simulink model "G24i_v_source"  (R2014a)
settings: Solver=ode23tb  StartTime=0.0  StopTime=5  RelTol=1e-4
values from neighbouring files (symbols this model uses):
  Array_Voc = [0.328644000009 2.76811 3.09396940822 3.26133568944 3.36629977409 3.44398192097 3.50365713438 3.55225637345 3.59363766529 3.63021764721 3.6624 3.69037314882 ... (101 elements, 101x1)]    [Array_Voc.mat]
  ArrayCurrent = [1.05303e-05 0.0329007487024 0.0659314357778 0.100205 0.132978217474 0.166891516648 0.200872978445 0.234107600227 0.267513340222 0.302009988541 0.336322 0.36979130469 ... (44440 elements, 101x440)]    [ArrayCurrent.mat]    (also in Genrate_SC_mod.m = fitresult_normal_g42(V,G); temp3.m = fitresult(V,G))
  ArrayVoltage = [0 0.01 0.02 0.03 0.04 0.05 0.06 0.07 0.08 0.09 0.1 0.11 ... (440 elements, 1x440)]    [ArrayVoltage.mat]    (also in Genrate_SC_mod.m = (0:0.01:max(Voltage)); temp3.m = (0:0.01:max(Voltage)))
  Irradiance = (min(Lux):50:max(Lux))    [Genrate_SC_mod.m]    (also in Irradiance.mat = [0 50 100 150 200 250 300 350 400 450 500 550 ... (101 eleme; temp3.m)
undefined symbols (not defined in the file or in its folder): sigbuilder_block
libraries: powerlib x7, simulink_extras x4
settings Model: NumberOfSteps=5  Creator=kartik.karuna  LastModifiedBy=kartik.karuna
settings SolverCC: SolverJacobianMethodControl=SparsePerturbation  ZeroCrossAlgorithm=Adaptive  AutoInsertRateTranBlk=on

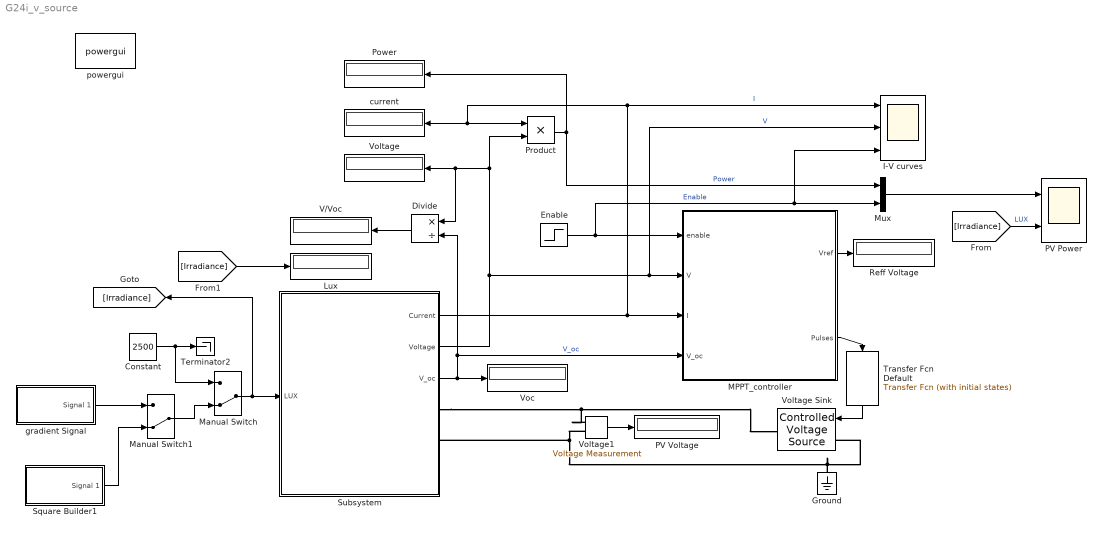
== system G24i_v_source ==
  Constant : Constant  Value=2500
  Divide : Product  Inputs=*/
  Enable : Step  Time=0.1  SampleTime=0
  Ground : powerlib/Elements/Ground  LConnTagsString=a
  I-V curves : Scope  NumInputPorts=3
      settings: ShowLegends=on  TimeRange=0.09  YMin=0.45~3.4875~1  YMax=0.8~3.5125~1
  Lux : Display
  MPPT_controller : Subsystem  Variant=on
  Manual Switch : ManualSwitch  CurrentSetting=0
  Manual Switch1 : ManualSwitch  CurrentSetting=0
  Mux : Mux  Inputs=2
  PV Power : Scope  NumInputPorts=2
      settings: ShowLegends=on  TimeRange=0.5  YMin=0~800  YMax=7~2000  SaveName=ScopeData2
  PV Voltage : Display
  Power : Display
  Product : Product  RndMeth=Zero
  Reff Voltage : Display
  Square Builder1 : Subsystem  Tag=STV Subsys  LoadFcn=sigbuilder_block('load');  StartFcn=sigbuilder_block('start');  StopFcn=sigbuilder_block('stop');  ClipboardFcn=sigbuilder_block('clipboard');  mask(Sigbuilder block){}
      mask help: Simulink:masks:SigbuilderBlock_MD
      mask init:
      | if ~strcmp(get_param(bdroot(gcbh),'SimulationStatus'),'stopped') tuvar = sigbuilder_block('maskInit'); end
      settings: CopyFcn=sigbuilder_block('copy');  DeleteFcn=sigbuilder_block('delete');  ModelCloseFcn=sigbuilder_block('modelClose');  PreSaveFcn=sigbuilder_block('preSave');  PauseFcn=sigbuilder_block('pause');  ContinueFcn=sigbuilder_block('continue');  NameChangeFcn=sigbuilder_block('namechange');  OpenFcn=sigbuilder_block('open',[0 29.7931 1588.97 810.621 ]);  CloseFcn=sigbuilder_block('close');
      mask Display: plot(0, 0, 100, 100,[2, 2, 32, 32, 2], [68, 8, 8, 68, 68],[32, 2], [38, 38], [32, 19, 2],[53, 60, 44], [32, 17, 17, 2],[16, 16, 31, 31]);txt = getActiveGroup(gcbh);text(2, 100, txt,'verticalAlignment', 'top');
  Subsystem : Subsystem
  Terminator2 : Terminator
  Transfer Fcn Default : simulink_extras/Additional Linear/Transfer Fcn (with initial states)  VariantControl=(default)  N=[1]  D="[.00001  1]"  X0=0
  V/Voc : Display
  Voc : Display
  Voltage : Display
  Voltage Sink : powerlib/Electrical Sources/Controlled Voltage Source  Initialize=on  Source_Type=AC  Amplitude=0  Phase=0  Frequency=0  Measurements=Voltage
  Voltage1 : powerlib/Measurements/Voltage Measurement  PhasorSimulation=off  OutputType=Complex  PSBequivalent=0
  current : Display
  gradient Signal : Subsystem  Tag=STV Subsys  LoadFcn=sigbuilder_block('load');  StartFcn=sigbuilder_block('start');  StopFcn=sigbuilder_block('stop');  ClipboardFcn=sigbuilder_block('clipboard');  mask(Sigbuilder block){}
      mask help: Simulink:masks:SigbuilderBlock_MD
      mask init:
      | if ~strcmp(get_param(bdroot(gcbh),'SimulationStatus'),'stopped') tuvar = sigbuilder_block('maskInit'); end
      settings: CopyFcn=sigbuilder_block('copy');  DeleteFcn=sigbuilder_block('delete');  ModelCloseFcn=sigbuilder_block('modelClose');  PreSaveFcn=sigbuilder_block('preSave');  PauseFcn=sigbuilder_block('pause');  ContinueFcn=sigbuilder_block('continue');  NameChangeFcn=sigbuilder_block('namechange');  OpenFcn=sigbuilder_block('open',[1588.97 178.759 1271.17 661.655 ]);  CloseFcn=sigbuilder_block('close');
      mask Display: plot(0, 0, 100, 100,[2, 2, 32, 32, 2], [68, 8, 8, 68, 68],[32, 2], [38, 38], [32, 19, 2],[53, 60, 44], [32, 17, 17, 2],[16, 16, 31, 31]);txt = getActiveGroup(gcbh);text(2, 100, txt,'verticalAlignment', 'top');
  powergui : powerlib/powergui  Priority=1  SimulationMode=Continuous  SolverType=Tustin  SampleTime=50e-6  frequency=50  SPID=off  DisableSnubberDevices=off  DisableRonSwitches=off  DisableVfSwitches=off  SwTol=0  Interpol=off  DisplayEquations=off  Ts=0  methode=off  frequencyindice=0  Pbase=100e6  ErrMax=1e-4  Iterations=50  UnitsV=kV  UnitsW=MW  FunctionMessages=off  echomessages=off  HookPort=off  EnableUseOfTLC=off  x0status=blocks  RestoreLinks=warning  ResistiveCurrentMeasurement=off  Frange=[0:2:500]  Ylog=off  Xlog=on  ShowGrid=off  save=off  variable=ZData  structure=0  ZoomFFT=off  StartTime=0.0  cycles=1  DisplayStyle=1  fundamental=60  FreqAxis=off  MaxFrequency=1000  frequencyindicesteady=1  RmsSteady=1  display=off
  wires:
  Mux/1 -> PV Power/1
  Product/1 -> Power/1, Mux/1  "Power"
  Voltage1/1 -> PV Voltage/1
  Enable/1 -> MPPT_controller/1(enable), I-V curves/3, Mux/2  "Enable"
  Subsystem/3("V_oc ") -> Divide/2, MPPT_controller/4(V_oc), Voc/1  "V_oc"
  Divide/1 -> V/Voc/1
  MPPT_controller/1(Vref) -> Reff Voltage/1
  Subsystem/2(Voltage) -> Divide/1, Voltage/1, Product/2, I-V curves/2, MPPT_controller/2(V)  "V"
  Subsystem/1(Current) -> I-V curves/1, current/1, Product/1, MPPT_controller/3(I)  "I"
  Constant/1 -> Manual Switch/1, Terminator2/1
  [Irradiance] -> PV Power/2  "LUX"
  Manual Switch/1 -> Subsystem/1(LUX), [Irradiance]
  [Irradiance] -> Lux/1
  Manual Switch1/1 -> Manual Switch/2
  gradient Signal/1(Signal 1) -> Manual Switch1/1
  Square Builder1/1(Signal 1) -> Manual Switch1/2
  MPPT_controller/2(Pulses) -> Transfer Fcn Default/1
  Transfer Fcn Default/1 -> Voltage Sink/1
  connections:
  Subsystem/RConn1 -- Voltage1/LConn1 -- Voltage Sink/RConn1
  Voltage1/LConn2 -- Voltage Sink/LConn1 -- Ground/LConn1 -- Subsystem/RConn2

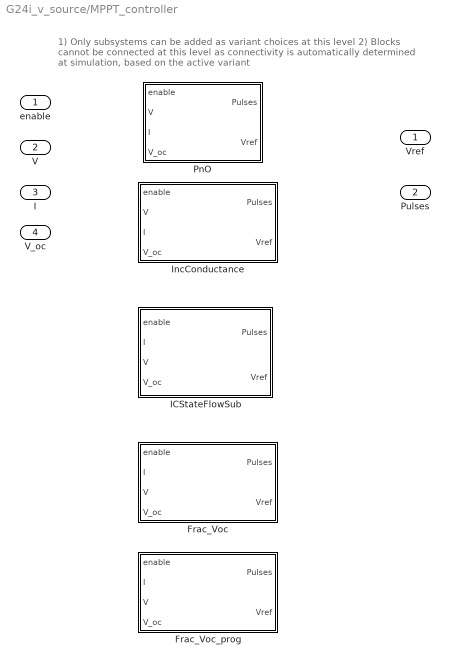
== system G24i_v_source/MPPT_controller ==
  note: 1) Only subsystems can be added as variant choices at this level
      | 2) Blocks cannot be connected at this level as connectivity is
      | automatically determined at simulation, based on the active variant
  enable : Inport
  V : Inport  Port=2
  I : Inport  Port=3
  V_oc : Inport  Port=4
  Frac_Voc : Subsystem  VariantControl=MPPT_Frac_Voc
  Frac_Voc_prog : Subsystem  VariantControl=MPPT_Frac_Voc_prog
  ICStateFlowSub : Subsystem  VariantControl=MPPT_IC_SF
  IncConductance : Subsystem  VariantControl=MPPT_IC_logic
  PnO : Subsystem  VariantControl=MPPT_PnO
  Vref : Outport
  Pulses : Outport  Port=2

== system G24i_v_source/Square Builder1 ==
  Demux : Demux  Tag=STV Demux  Outputs=1
  FromWs : FromWorkspace  Tag=STV FromWs  VariableName=tuvar  SampleTime=0
      SigBuilderData=|
      | common.afterFinalStr = 'Extrapolate'
      | common.sampleTime = 0
      | dataSet.timeRange = [0 2]
      | dataSet.name = 'Group 1'
      | sbobj.Groups.Name = 'Group 1'
      | sbobj.Groups.Signals.Name = 'Signal 1'
      | sbobj.Groups.Signals.XData = [0 0.3 0.4 0.4 0.6 0.6 0.6 0.7 0.7 0.8 0.8 1.1 1.1 1.2 1.2 1.4 1.4 1.8 1.8 1.9 2]
      | sbobj.Groups.Signals.YData = [2500 2500 2500 2000 2000 1500 1500 1500 1000 1000 800 800 1200 1200 1500 1500 1000 1000 400 400 400]
      | sbobj.Groups.TimeRange = [0 2]
  Signal 1 : Outport  Tag=STV Outport
  wires:
  FromWs/1 -> Demux/1
  Demux/1 -> Signal 1/1

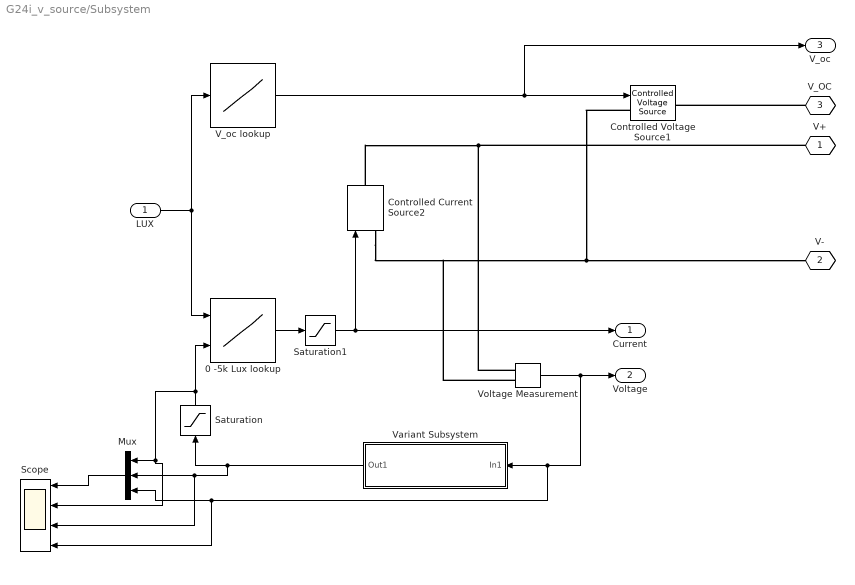
== system G24i_v_source/Subsystem ==
  LUX : Inport
  0 -5k Lux lookup : Lookup_n-D  BreakpointsForDimension1=Irradiance  BreakpointsForDimension2=ArrayVoltage  BreakpointsForDimension1Min=[0]  BreakpointsForDimension2Min=[0]  BreakpointsForDimension1Max=[5000]  BreakpointsForDimension2Max=[6]  Table=ArrayCurrent  DiagnosticForOutOfRangeInput=Warning  RndMeth=Simplest  InputSameDT=on
  Controlled Current Source2 : powerlib/Electrical Sources/Controlled Current Source  Initialize=on  Source_Type=DC  Amplitude=0  Phase=0  Frequency=0  Measurements=None
  Controlled Voltage Source1 : powerlib/Electrical Sources/Controlled Voltage Source  Initialize=on  Source_Type=AC  Amplitude=0  Phase=0  Frequency=0  Measurements=Voltage
  Mux : Mux  Inputs=3
  Saturation : Saturate  UpperLimit=6  LowerLimit=0  ZeroCross=off
  Saturation1 : Saturate  UpperLimit=6  LowerLimit=-1
  Scope : Scope  NumInputPorts=4
      settings: YMin=-5~-5~-5~-5  YMax=5~5~5~5
  V_oc lookup : Lookup_n-D  NumberOfTableDimensions=1  BreakpointsForDimension1=Irradiance  Table=Array_Voc  RndMeth=Simplest  InputSameDT=on
  Variant Subsystem : Subsystem  Variant=on
  Voltage Measurement : powerlib/Measurements/Voltage Measurement  PhasorSimulation=off  OutputType=Complex  PSBequivalent=0
  V+ : PMIOPort  Tag=PMCPort  Port=1  Side=Right
  V- : PMIOPort  Tag=PMCPort  Port=2  Side=Right
  V_OC : PMIOPort  Tag=PMCPort  Port=3  Side=Right
  Current : Outport
  Voltage : Outport  Port=2
  "V_oc " : Outport  Port=3
  wires:
  LUX/1 -> 0 -5k Lux lookup/1, V_oc lookup/1
  Voltage Measurement/1 -> Voltage/1, Scope/4, Mux/3, Variant Subsystem/1(In1)
  0 -5k Lux lookup/1 -> Saturation1/1
  V_oc lookup/1 -> "V_oc "/1, Controlled Voltage Source1/1
  Saturation/1 -> 0 -5k Lux lookup/2, Scope/2, Mux/1
  Saturation1/1 -> Controlled Current Source2/1, Current/1
  Mux/1 -> Scope/1
  Variant Subsystem/1(Out1) -> Scope/3, Mux/2, Saturation/1
  connections:
  Controlled Current Source2/RConn1 -- V+/RConn1 -- Voltage Measurement/LConn1
  Controlled Voltage Source1/LConn1 -- Voltage Measurement/LConn2 -- Controlled Current Source2/LConn1 -- V-/RConn1
  V_OC/RConn1 -- Controlled Voltage Source1/RConn1

== system G24i_v_source/gradient Signal ==
  Demux : Demux  Tag=STV Demux  Outputs=1
  FromWs : FromWorkspace  Tag=STV FromWs  VariableName=tuvar  SampleTime=0
      SigBuilderData=|
      | common.afterFinalStr = 'Extrapolate'
      | common.sampleTime = 0
      | dataSet.timeRange = [0 2]
      | dataSet.name = 'Group 1'
      | sbobj.Groups.Name = 'Group 1'
      | sbobj.Groups.Signals.Name = 'Signal 1'
      | sbobj.Groups.Signals.XData = [0 0.35 0.55 0.85 1.2 2]
      | sbobj.Groups.Signals.YData = [2500 2500 200 200 800 800]
      | sbobj.Groups.TimeRange = [0 2]
  Signal 1 : Outport  Tag=STV Outport
  wires:
  Demux/1 -> Signal 1/1
  FromWs/1 -> Demux/1

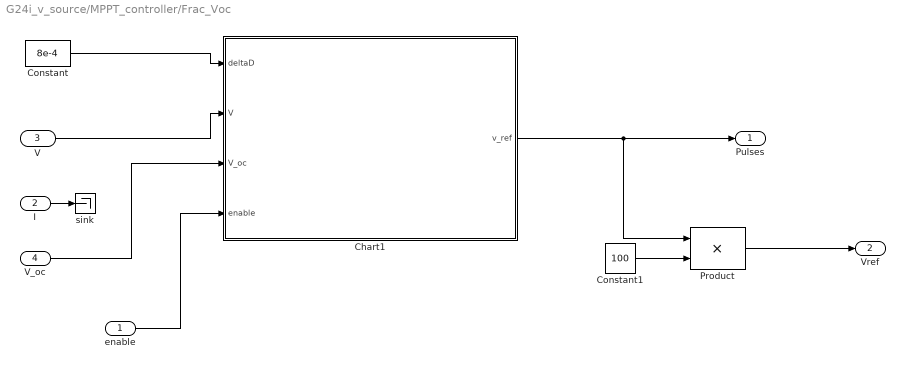
== system G24i_v_source/MPPT_controller/Frac_Voc ==
  enable : Inport
  I : Inport  Port=2
  V : Inport  Port=3
  V_oc : Inport  Port=4
  Chart1 : Stateflow chart  TreatAsAtomicUnit=on
  Constant : Constant  Value=8e-4
  Constant1 : Constant  Value=100
  Product : Product  RndMeth=Zero
  sink : Terminator
  Pulses : Outport
  Vref : Outport  Port=2
  wires:
  Constant/1 -> Chart1/1(deltaD)
  V/1 -> Chart1/2(V)
  enable/1 -> Chart1/4(enable)
  Chart1/1(v_ref) -> Pulses/1, Product/1
  Constant1/1 -> Product/2
  Product/1 -> Vref/1
  V_oc/1 -> Chart1/3(V_oc)
  I/1 -> sink/1

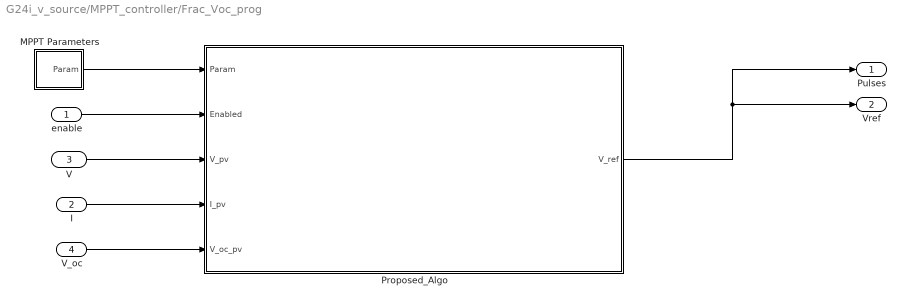
== system G24i_v_source/MPPT_controller/Frac_Voc_prog ==
  enable : Inport
  I : Inport  Port=2
  V : Inport  Port=3
  V_oc : Inport  Port=4
  MPPT Parameters : Subsystem
  Proposed_Algo : MATLAB Function  TreatAsAtomicUnit=on
  Pulses : Outport
  Vref : Outport  Port=2
  wires:
  I/1 -> Proposed_Algo/4(I_pv)
  MPPT Parameters/1(Param) -> Proposed_Algo/1(Param)
  enable/1 -> Proposed_Algo/2(Enabled)
  V/1 -> Proposed_Algo/3(V_pv)
  V_oc/1 -> Proposed_Algo/5(V_oc_pv)
  Proposed_Algo/1(V_ref) -> Pulses/1, Vref/1

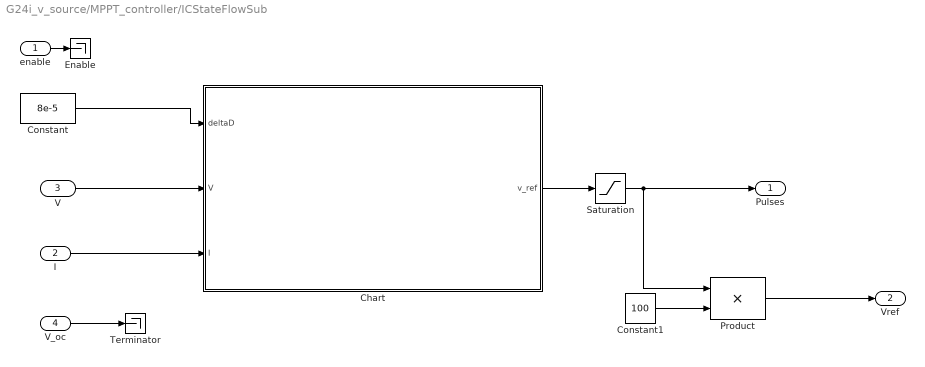
== system G24i_v_source/MPPT_controller/ICStateFlowSub ==
  enable : Inport
  I : Inport  Port=2
  V : Inport  Port=3
  V_oc : Inport  Port=4
  Chart : Stateflow chart  TreatAsAtomicUnit=on
  Constant : Constant  Value=8e-5
  Constant1 : Constant  Value=100
  "Enable " : Terminator
  Product : Product  RndMeth=Zero
  Saturation : Saturate  UpperLimit=.95  LowerLimit=0.1
  Terminator : Terminator
  Pulses : Outport
  Vref : Outport  Port=2
  wires:
  I/1 -> Chart/3(I)
  Constant/1 -> Chart/1(deltaD)
  V/1 -> Chart/2(V)
  enable/1 -> "Enable "/1
  Chart/1(v_ref) -> Saturation/1
  Saturation/1 -> Pulses/1, Product/1
  Constant1/1 -> Product/2
  Product/1 -> Vref/1
  V_oc/1 -> Terminator/1

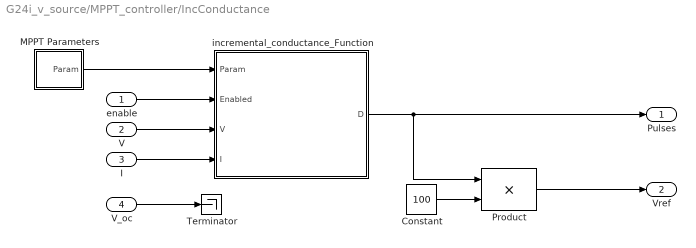
== system G24i_v_source/MPPT_controller/IncConductance ==
  enable : Inport
  V : Inport  Port=2
  I : Inport  Port=3
  V_oc : Inport  Port=4
  Constant : Constant  Value=100
  MPPT Parameters : Subsystem
  Product : Product  RndMeth=Zero
  Terminator : Terminator
  "incremental_conductance_Function " : MATLAB Function  TreatAsAtomicUnit=on
  Pulses : Outport
  Vref : Outport  Port=2
  wires:
  V/1 -> "incremental_conductance_Function "/3(V)
  I/1 -> "incremental_conductance_Function "/4(I)
  Constant/1 -> Product/2
  Product/1 -> Vref/1
  "incremental_conductance_Function "/1(D) -> Pulses/1, Product/1
  enable/1 -> "incremental_conductance_Function "/2(Enabled)
  V_oc/1 -> Terminator/1
  MPPT Parameters/1(Param) -> "incremental_conductance_Function "/1(Param)

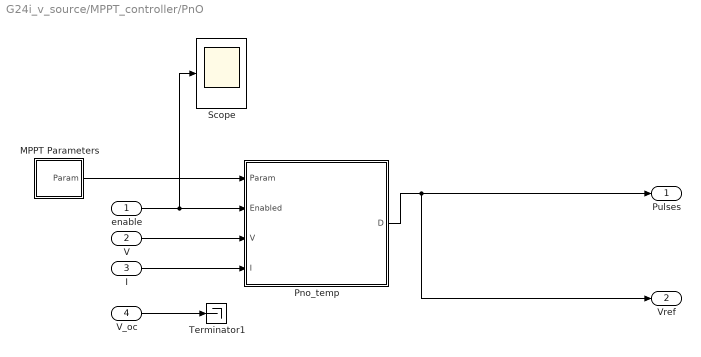
== system G24i_v_source/MPPT_controller/PnO ==
  enable : Inport
  V : Inport  Port=2
  I : Inport  Port=3
  V_oc : Inport  Port=4
  MPPT Parameters : Subsystem
  Pno_temp : MATLAB Function  TreatAsAtomicUnit=on
      settings: MinAlgLoopOccurrences=on
  Scope : Scope
      settings: TimeRange=1  YMin=-4.16334e-17  YMax=0.6  SaveName=ScopeData4
  Terminator1 : Terminator
  Pulses : Outport
  Vref : Outport  Port=2
  wires:
  enable/1 -> Pno_temp/2(Enabled), Scope/1
  V_oc/1 -> Terminator1/1
  MPPT Parameters/1(Param) -> Pno_temp/1(Param)
  V/1 -> Pno_temp/3(V)
  I/1 -> Pno_temp/4(I)
  Pno_temp/1(D) -> Vref/1, Pulses/1

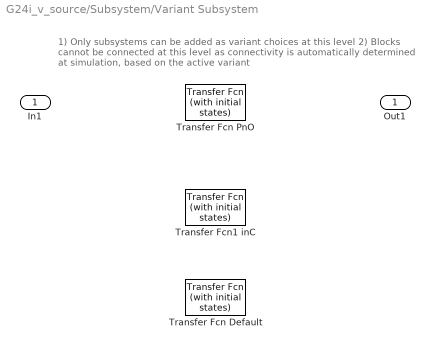
== system G24i_v_source/Subsystem/Variant Subsystem ==
  note: 1) Only subsystems can be added as variant choices at this level
      | 2) Blocks cannot be connected at this level as connectivity is
      | automatically determined at simulation, based on the active variant
  In1 : Inport
  Transfer Fcn Default : simulink_extras/Additional Linear/Transfer Fcn (with initial states)  VariantControl=(default)  N=[1]  D="[.001  1]"  X0=0
  Transfer Fcn PnO : simulink_extras/Additional Linear/Transfer Fcn (with initial states)  VariantControl=MPPT_PnO  N=[1]  D="[.0001  1]"  X0=0
  Transfer Fcn1 inC : simulink_extras/Additional Linear/Transfer Fcn (with initial states)  VariantControl=MPPT_IC_logic  N=[1]  D="[.001  1]"  X0=0
  Out1 : Outport

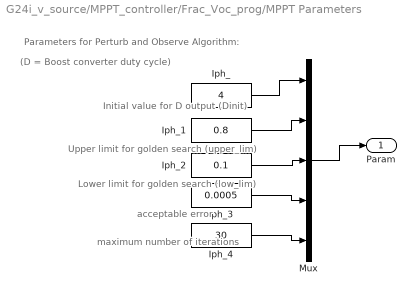
== system G24i_v_source/MPPT_controller/Frac_Voc_prog/MPPT Parameters ==
  note: Upper limit for golden search (upper_lim)
  note: maximum number of iterations
  note: Initial value for D output (Dinit)
  note: (D = Boost converter duty cycle)
  note: Lower limit for golden search (low_lim)
  note: Parameters for Perturb and Observe Algorithm:
  note: acceptable error
  Iph_ : Constant  Value=4
  Iph_1 : Constant  Value=0.8
  Iph_2 : Constant  Value=0.1
  Iph_3 : Constant  Value=0.0005
  Iph_4 : Constant  Value=30
  Mux : Mux  Inputs=5
  Param : Outport
  wires:
  Iph_/1 -> Mux/1
  Iph_1/1 -> Mux/2
  Iph_2/1 -> Mux/3
  Iph_3/1 -> Mux/4
  Mux/1 -> Param/1
  Iph_4/1 -> Mux/5

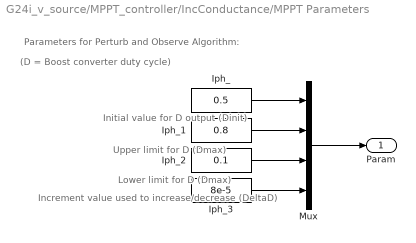
== system G24i_v_source/MPPT_controller/IncConductance/MPPT Parameters ==
  note: Upper limit for D (Dmax)
  note: Increment value used to increase/decrease (DeltaD)
  note: Initial value for D output (Dinit)
  note: (D = Boost converter duty cycle)
  note: Lower limit for D (Dmax)
  note: Parameters for Perturb and Observe Algorithm:
  Iph_ : Constant  Value=0.5
  Iph_1 : Constant  Value=0.8
  Iph_2 : Constant  Value=0.1
  Iph_3 : Constant  Value=8e-5
  Mux : Mux
  Param : Outport
  wires:
  Iph_/1 -> Mux/1
  Iph_1/1 -> Mux/2
  Iph_2/1 -> Mux/3
  Iph_3/1 -> Mux/4
  Mux/1 -> Param/1

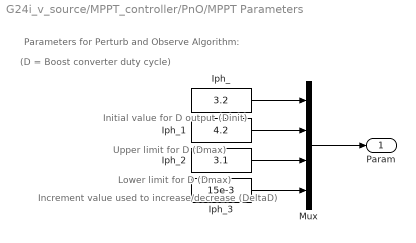
== system G24i_v_source/MPPT_controller/PnO/MPPT Parameters ==
  note: Upper limit for D (Dmax)
  note: Increment value used to increase/decrease (DeltaD)
  note: Initial value for D output (Dinit)
  note: (D = Boost converter duty cycle)
  note: Lower limit for D (Dmax)
  note: Parameters for Perturb and Observe Algorithm:
  Iph_ : Constant  Value=3.2
  Iph_1 : Constant  Value=4.2
  Iph_2 : Constant  Value=3.1
  Iph_3 : Constant  Value=15e-3
  Mux : Mux
  Param : Outport
  wires:
  Iph_/1 -> Mux/1
  Iph_1/1 -> Mux/2
  Iph_2/1 -> Mux/3
  Iph_3/1 -> Mux/4
  Mux/1 -> Param/1

== matlab function G24i_v_source/MPPT_controller/IncConductance/incremental_conductance_Function  ==
  settings: updateMethod=DISCRETE  sampleTime=Ts_Control
  data: Param input; Enabled input; V input; I input; D output
function D  = IncC_Pog(Param, Enabled, V, I)
% MPPT controller block based on the incremental conductance algorithm
% MPPT controller based on the Perturb & Observe algorithm.

% D output = Duty cycle  (value between 0 and 1)
%
% Enabled input = 1 to enable the MPPT controller
% V input = PV array terminal voltage (V)
% I input = PV array current (A)
%
% Param input:
Dinit = Param(1);  %Initial value for D output
Dmax = Param(2);   %Maximum value for D
Dmin = Param(3);   %Minimum value for D
deltaD = Param(4); %Increment value used to increase/decrease the duty cycle D

% ( increasing D = decreasing Vref )
persistent Vold Dold Iold;

dataType = 'double';

if isempty(Vold)
    Vold=0;
    Iold=0;
    Dold=Dinit;
    D=Dinit;
    
end

dV= V - Vold;
dI= I- Iold;


if Enabled == 1
   if dV==0
       if dI ~= 0
           if dI >0
               D = Dold + deltaD;
           else 
               D = Dold + deltaD;
           end
       else
           D=Dold;
       end
       Dold=D;
       Vold=V;
       Iold=I;
   else
       if ((dI/dV) ~= (-I/V))
           if ((dI/dV) > (-I/V))
               D = Dold - deltaD;
           else 
               D = Dold + deltaD;
           end
       else
           D=Dold;
       end
       Dold=D;
       Vold=V;
       Iold=I;
   end
  
else
    D=Dold;
end

if D >= Dmax | D<= Dmin
    D=Dold;
end

== matlab function G24i_v_source/MPPT_controller/Frac_Voc_prog/Proposed_Algo ==
  data: Param input; V_ref output; Enabled input; V_pv input; I_pv input; V_oc_pv input
function V_ref   = cyrx_prop(Param, Enabled, V_pv,I_pv, V_oc_pv)

% MPPT controller based on algorithm proposed by Kartik Karuna for his
% Exjobb at Exeger Sweden AB 

% V_ref = reference voltage for DC converter 

% Enabled input = 1 to enable the MPPT controller
% V input = PV array terminal voltage (V)
% I input = PV array current (A)
% V_oc    = Open circuit Voltage of the PV array
% Param input:

Dinit = Param(1);  %Initial value for D output

error= Param(4);          %Increment value used to increase/decrease the duty cycle D
iteration_lim= Param(5);  % maximum number of iterations
tau=double((sqrt(5)-1)/2);
rsq_min = 0.87;
% ( increasing D = decreasing Vref )

cons = zeros(1,2);
persistent  Dold Voc_old upper_lim low_lim iteration_count flag Xs Vs idx done;


dataType = 'double';

% for the first time the program is run
if isempty(Dold)
      Dold=Dinit;
      Voc_old=0;
      iteration_count=0;
      upper_lim = Param(2); % end of interval
      low_lim = Param(3);   % start of interval default value
      flag =0;
      Xs=zeros(2,2); %[x1,f_fx1:x2,f_x2]
      Vs=zeros(20,2);%[voc:Vmpp]
      idx=1;
      done=0;
end
% Load look up table from memory calculate constants for the line y = mx+b 
%look_up=load('look_up_line_eq.mat','voc','vmpp','idx','x1','x2');

% if any of the voc or vmpp values are '0' then the array is not yet full
% and not yet ready to be used.
V_ref=Dold;

if Enabled == 1
   % check if value of v_oc has changed

   if (abs(Voc_old-V_oc_pv)>0.002||done==0)
       
       
       if done==1
       
           flag =0; % measure xs and Fxs
           Xs(1,2)=0;
           Xs(2,2)=0;
       end    
       done=0;
        %% Line regression      
        if (iteration_count==0) %% check
            cons(1)=0.9586;
            cons(2)=-0.5409;
            % if Look up table is not yet populated.
            if (any(Vs(:,1)==0) || any(Vs(:,2)==0))
                %do nothing
            else    
                cons_t = polyfit( Vs(:,1),Vs(:,2),1);
                % calculate the value of R^2
                yfit = polyval(cons_t,Vs(:,1));
                yresid = Vs(:,2) - yfit;
                SSresid = sum(yresid.^2);
                SStotal = (length(Vs(:,2))-1) * var(Vs(:,2));
                rsq = 1 - SSresid/SStotal;
                % use regression value only if r^2 better that 0.87
                if rsq > rsq_min
                cons = cons_t;
                end
            end
            prelim_mpp=((cons(1))*V_oc_pv)+cons(2);
            upper_lim=prelim_mpp+0.4;
            low_lim  =   prelim_mpp-0.5;
        end
        %Vmpp = ((cons(1))*V_oc_pv)+cons(2);
        %% Golden Search 
        Xs(1,1)=low_lim+(1-tau)*(upper_lim-low_lim); %x1
        Xs(2,1)=low_lim+tau*(upper_lim-low_lim);     %x2
        
        
        if((abs(low_lim-upper_lim)>error)&&iteration_count<iteration_lim&&flag>2)
         
            if(Xs(1,2)>Xs(2,2))
                upper_lim=Xs(2,1);
                Xs(2,1)=Xs(1,1);
                Xs(1,1)=low_lim+(1-tau)*(upper_lim-low_lim);
                %Cal f_X for both
                flag =0
            else
                low_lim=Xs(1,1);
                Xs(1,1)=Xs(2,1);
                Xs(2,1)=low_lim+tau*(upper_lim-low_lim);
                %Cal f_X for both
                flag =0
            end
            iteration_count=iteration_count+1        
        elseif(((abs(low_lim-upper_lim)<error)||iteration_count>=iteration_lim)&&(flag>2))
            iteration_count
            iteration_count=0;
            done=1;
            Vs(idx,1)=V_oc_pv;
            Vs(idx,2)=V_pv;
            idx=idx+1;
            if idx==20
                idx=1;
            end    
        end
        
        %Compute F_x1 and F_x2        
        if flag==0
              figure(1)
            hold all;
           V_ref=Xs(1,1);      %x1
           flag=1;
        elseif flag==1
           Xs(1,2)=V_pv*I_pv    %f_x1
           V_ref= Xs(2,1);      %x2
           flag =2;
           
            plot(low_lim,1,'b*');
        elseif flag==2
           Xs(2,2)=V_pv*I_pv    %f_x2
           flag=3;
           plot(upper_lim,1,'r*');
            hold on
            
        end
       
   
   end

  
   Voc_old=V_oc_pv;
end

Dold=V_ref;

== stateflow chart G24i_v_source/MPPT_controller/ICStateFlowSub/Chart ==
  state init
    entry:
    V_prev1=0;
    I_prev1=0;
    V_REF=0.5;
  state Sample_and_call
    entry:
    deltaV = V -V_prev1;
    deltaI = I - I_prev1;
    v_ref = V_REF;
  state INCREMENT
    entry:
    v_ref =v_ref+deltaD;
  state DECREMENT
    entry:
    v_ref =v_ref-deltaD;
  state RETURN
    entry:
    V_prev1 = V;
    I_prev1 = I ;
    V_REF= v_ref;
  (default) -> init
  init -> Sample_and_call
  RETURN -> Sample_and_call
  Sample_and_call -> (junction 35)
  (junction 35) -> (junction 6) [order 2] : [deltaV==0]
  (junction 35) -> (junction 22) [order 1] : [deltaV~=0]
  (junction 6) -> RETURN [order 2] : [deltaI==0]
  (junction 6) -> (junction 16) [order 1] : [deltaI~=0]
  (junction 22) -> RETURN [order 2] : [deltaI/deltaV == -(I/V)]
  (junction 22) -> (junction 15) [order 1] : [deltaI/deltaV ~= -(I/V)]
  (junction 16) -> DECREMENT [order 2] : [deltaI<=0]
  (junction 16) -> INCREMENT [order 1] : [deltaI>0]
  (junction 15) -> INCREMENT [order 2]
  (junction 15) -> DECREMENT [order 1] : [(deltaI/deltaV) > -(I/V)]
  INCREMENT -> RETURN
  DECREMENT -> RETURN
  data: deltaD input; v_ref output double; V_prev1 local =0; I_prev1 local =0; V_REF local =0; deltaV local; deltaI local; V input; I input

== stateflow chart G24i_v_source/MPPT_controller/Frac_Voc/Chart1 ==
  state init
    entry:
    V_REF=0.5;
    Vmpp=(0.9501)*(V_oc)-(0.4825);
  state Sample_and_call
    entry:
    deltaV = V -Vmpp;
    v_ref=Vmpp;;
  Sample_and_call -> init
  (default) -> init
  init -> Sample_and_call : [enable > 0]
  data: deltaD input; Vmpp local; deltaV local; v_ref output; V_REF local; V input; V_oc input; enable input

== matlab function G24i_v_source/MPPT_controller/PnO/Pno_temp ==
  data: Param input; D output; Enabled input; V input; I input
function D  = PandO(Param, Enabled, V, I)

% MPPT controller based on the Perturb & Observe algorithm.

% D output = Duty cycle  (value between 0 and 1)
%
% Enabled input = 1 to enable the MPPT controller
% V input = PV array terminal voltage (V)
% I input = PV array current (A)
%
% Param input:
Dinit = Param(1);  %Initial value for D output
Dmax = Param(2);   %Maximum value for D
Dmin = Param(3);   %Minimum value for D
deltaD = Param(4); %Increment value used to increase/decrease the duty cycle D
% ( increasing D = decreasing Vref )


persistent Vold Pold Dold;

dataType = 'double';

if isempty(Vold)
    Vold=0;
    Pold=0;
    Dold=Dinit;
end
P= V*I;
dV= V - Vold;
dP= P - Pold;

if dP ~= 0 & Enabled ~=0
    if dP < 0
        if dV < 0
            D = Dold - deltaD;
        else
            D = Dold + deltaD;
        end
    else
        if dV < 0
            D = Dold + deltaD;
        else
            D = Dold - deltaD;
        end    
    end
else D=Dold;
end

if D >= Dmax | D<= Dmin
    D=Dold;
end

Dold=D;
Vold=V;
Pold=P;
